simulink model "testSignalBuilder"  (R2018a)
settings: Solver=VariableStepAuto  StartTime=0.0  StopTime=10  RelTol=1e-3
undefined symbols (not defined in the file): sigbuilder_block
settings Model: Creator=BEAR  LastModifiedBy=BEAR

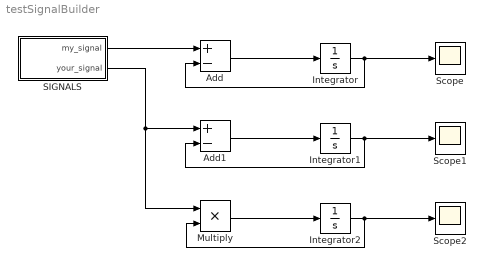
== system testSignalBuilder ==
  Add : Sum  Inputs=+-
  Add1 : Sum  Inputs=+-
  Integrator : Integrator
  Integrator1 : Integrator
  Integrator2 : Integrator  InitialCondition=1
  Multiply : Product
  SIGNALS : Subsystem  Tag=STV Subsys  LoadFcn=sigbuilder_block('load');  StartFcn=sigbuilder_block('start');  StopFcn=sigbuilder_block('stop');  ClipboardFcn=sigbuilder_block('clipboard');  mask(Sigbuilder block){tuvar=[0:10]}
      mask help: Simulink:masks:SigbuilderBlock_MD
      mask init:
      | if ~strcmp(get_param(bdroot(gcbh),'SimulationStatus'),'stopped') tuvar = sigbuilder_block('maskInit'); end
      settings: CopyFcn=sigbuilder_block('copy');  DeleteFcn=sigbuilder_block('delete');  ModelCloseFcn=sigbuilder_block('modelClose');  PreSaveFcn=sigbuilder_block('preSave');  PauseFcn=sigbuilder_block('pause');  ContinueFcn=sigbuilder_block('continue');  NameChangeFcn=sigbuilder_block('namechange');  OpenFcn=sigbuilder_block('open',[0 68 1280 636 ]);  CloseFcn=sigbuilder_block('close');
      mask Display: plot(0, 0, 100, 100,[2, 2, 32, 32, 2], [68, 8, 8, 68, 68],[32, 2], [38, 38], [32, 19, 2],[53, 60, 44], [32, 17, 17, 2],[16, 16, 31, 31]);txt = getActiveGroup(gcbh);text(2, 100, txt,'verticalAlignment', 'top');
  Scope : Scope
  Scope1 : Scope
  Scope2 : Scope
  wires:
  Add/1 -> Integrator/1
  Integrator/1 -> Scope/1, Add/2
  Add1/1 -> Integrator1/1
  Integrator1/1 -> Scope1/1, Add1/2
  SIGNALS/1(my_signal) -> Add/1
  SIGNALS/2(your_signal) -> Multiply/1, Add1/1
  Multiply/1 -> Integrator2/1
  Integrator2/1 -> Multiply/2, Scope2/1

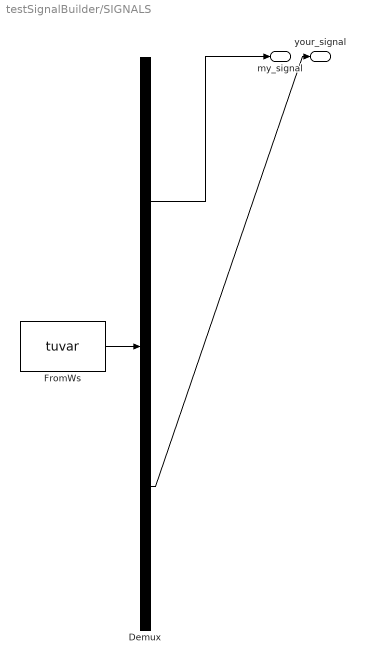
== system testSignalBuilder/SIGNALS ==
  Demux : Demux  Tag=STV Demux  Outputs=2
  FromWs : FromWorkspace  Tag=STV FromWs  VariableName=tuvar  SampleTime=0
      SigBuilderData=|
      | common.afterFinalStr = 'Extrapolate'
      | common.sampleTime = 0
      | dataSet.timeRange = [0 10]
      | dataSet.name = 'Group 1'
      | sbobj.Groups.Name = 'Group 1'
      | sbobj.Groups.Signals(1).Name = 'my_signal'
      | sbobj.Groups.Signals(1).XData = [0 1 2 3 4 5 6 7 8 9 10]
      | sbobj.Groups.Signals(1).YData = [0 1 0 -1 0 2 0 -2 0 -0.5 -0.5]
      | sbobj.Groups.Signals(2).Name = 'your_signal'
      | sbobj.Groups.Signals(2).XData = [0 1.5 1.5 4 4 6 6 8 8 9.5 9.5 10]
      | sbobj.Groups.Signals(2).YData = [0 0 -1 -1 1 1 0 0 -0.5 -0.5 0 0]
  my_signal : Outport  Tag=STV Outport
  your_signal : Outport  Tag=STV Outport  Port=2
  wires:
  Demux/1 -> my_signal/1
  FromWs/1 -> Demux/1
  Demux/2 -> your_signal/1
